simulink model "CML_Utility_Test"  (R2015a)
settings: Solver=ode4  SolverMode=MultiTasking  StartTime=0.0  StopTime=inf  FixedStep=BKIN_STEP_TIME  RelTol=1e-3
StartFcn:
  |  warndlg('Dexterit-E models cannot run under simulation. Please compile your model and run it from within Dexterit-E.');set_param(bdroot,'SimulationCommand','stop')
model workspace (MAT data in the model file):
  BKIN_STEP_TIME = 0.00025
  col_x = 1
  col_y = 2
  E_STAY_CENTER = 2
  INIT_COLOR = 5
  START_TARGET = 2
  MAX_REACH_TIME = 11
  DELAY_POST_TRIAL = 12
  BKIN_KINEMATIC_FRAME_SIZE = 400
  E_NO_EVENT = 0
  CHOICE_COLOR = 6
  FIXED_TARGET = 3
  FIXED_TARGET_VAL = 4
  GAMBLE_TARGET = 5
  GAMBLE_TARGET_VAL1 = 6
  GAMBLE_TARGET_VAL2 = 7
  DELAY_TARGET_FIXED = 8
  DELAY_TARGET_RANDOM = 9
  VWIDTH = 3
  VHEIGHT = 4
  TEXT = 8
  TEXT_COLOR = 9
  TEXT_HEIGHT = 10
  STROKE = 7
  TARGET_HOLD_TIME = 10
  E_HOLD_AT_FIXED_TARGET = 5
  E_HOLD_AT_GAMBLE_TARGET = 6
  K_SCORE_TARGET = 1
  E_CHOICES_ON = 3
  TRIAL_TYPE = 1
  E_PAUSE = 30
  E_EOT = 10
  CONTINUE = 2
  DELAY_CHOICE = 13
  E_WAIT = 4
  E_GO_TONE = 7
libraries: Video x4, General x3, slrtlib x3, KINARM_IO x2, KINARM_general x2, xpcnilib x2, simulink x1
CloseFcn:
  | rtwprivate ssgencode ModelCloseRequest b2lab2d
settings Model: ModifiedComment=chris -- Wed Feb 16 09:18:30 2005 -- Version 1.1384  ExtModeArmWhenConnect=off  ExtModeLogAll=off  LastModifiedBy=User
settings SolverCC: EnableConcurrentExecution=on  AutoInsertRateTranBlk=on
settings DataIOCC: LimitDataPoints=off  SignalLoggingSaveFormat=ModelDataLogs  SaveOutput=off  SaveTime=off  SignalLoggingName=sigsOut
settings OptimizationCC: BlockReduction=off  BooleanDataType=off  OptimizeBlockIOStorage=off  BufferReuse=off  GlobalBufferReuse=off  ExpressionFolding=off  ExpressionDepthLimit=2147483647  LocalBlockOutputs=off  InitFltsAndDblsToZero=on
settings DebuggingCC: SaveWithParameterizedLinksMsg=none  UnderspecifiedInitializationDetection=Classic  MergeDetectMultiDrivingBlocksExec=none  SignalResolutionControl=TryResolveAllWithWarning  MultiTaskDSMMsg=warning  FcnCallInpInsideContextMsg=UseLocalSettings  StateNameClashWarn=warning  StrictBusMsg=ErrorOnBusTreatedAsVector
settings HardwareCC: ProdIntDivRoundTo=Zero  ProdEndianess=LittleEndian  ProdLongLongMode=on  ProdHWDeviceType=Generic->32-bit x86 compatible  TargetHWDeviceType=32-bit Generic
settings SFSimCC: SimCustomHeaderCode="#include \"stdlib.h\""  SFSimEcho=off  SimParseCustomCode=off
settings RTWCC: SystemTargetFile=slrt.tlc  TemplateMakefile=slrt_default_tmf  Description=Simulink Real-Time  CustomSourceCode="#include \"stdlib.h\""  RTWCompilerOptimization=on
settings CodeAppCC: MaxIdLength=63
settings SimulinkRealTimeCC: TargetFcnLib=ansi_tfl_tmw.mat  GeneratePreprocessorConditionals=Disable all  xPCisDownloadable=off  xPCisDefaultEnv=off

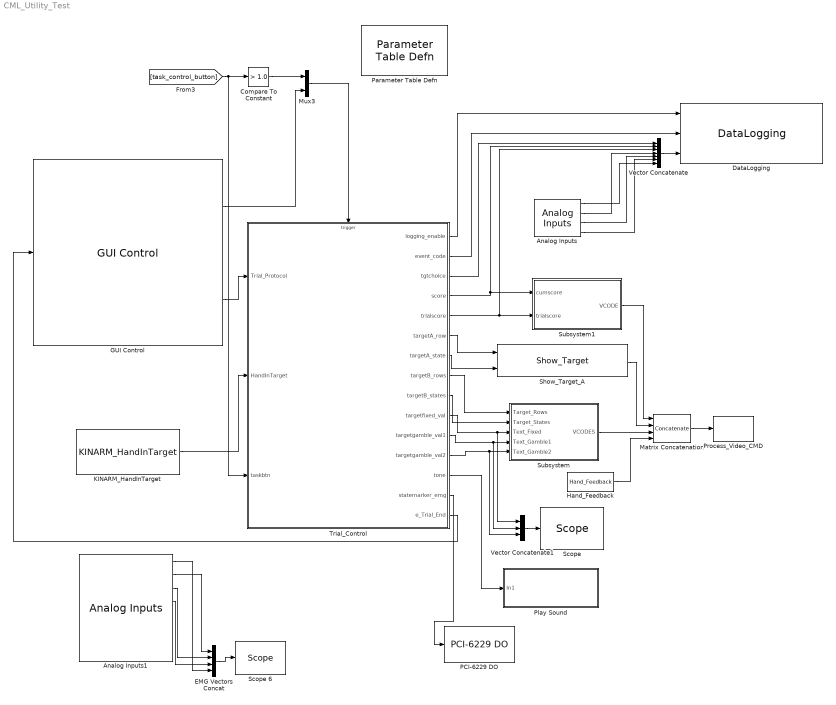
== system CML_Utility_Test ==
  Analog Inputs : KINARM_IO/Analog Inputs  channel=[17:20]  range=5  coupling=[0]  scantime6071e=1.28e-5  scantime6229=5e-6  sampletime=0.001  slot=-1  oscantime6071e=0
  Analog Inputs1 : KINARM_IO/Analog Inputs  channel=[17:24]  range=5  coupling=[0]  scantime6071e=1.28e-5  scantime6229=5e-6  sampletime=0.001  slot=-1  oscantime6071e=0
  Compare To Constant : simulink/Logic and Bit Operations/Compare To Constant  relop=>  const=1.0  OutDataTypeStr=boolean
  DataLogging : General/DataLogging  log_event_codes=on  log_analog_inputs=on  show_time_remaining=off  ecat_include=on
  EMG Vectors Concat : Concatenate  NumInputs=4
  GUI Control : General/GUI Control  task_version=1.0  show_repeat_trial_flag=off  use_custom_tp=off  target_type_str=Circle  Target_Type=1  XYcols=[1 2]  Vcols=3  Lcols=4  indices_padding=[0 0 0 0;0 0 0 0]  target_table_rows=64  load_table_rows=20  tp_table_rows=100
  Hand_Feedback : KINARM_general/Hand_Feedback  feedback_cntl_src=none
  KINARM_HandInTarget : KINARM_general/KINARM_HandInTarget  use_dominant_hand=on  target_type=Circle  num_states=1  attribcol1=[VWIDTH]  attribcol2=[0]  attribcol3=[0]  attribcol4=[0]  attribcol5=[0]
  Matrix Concatenation : Concatenate  NumInputs=4  Mode=Multidimensional array
  Mux3 : Mux  Inputs=2
  PCI-6229 DO : xpcnilib/Digital Output/M Series/PCI-6229 DO  channel=13  reset=[1]  initValue=[0]  sampletime=0.001  slot=-1
  Parameter Table Defn : General/Parameter Table Defn  ShowInLibBrowser=0
  Play Sound : Subsystem
  Process_Video_CMD : Video/Process_Video_CMD  video_delay=0
  "Scope " : slrtlib/Displays and Logging/Scope   scopeno=2  scopetype=Target  autostart=on  viewmode=Numerical  formatstr='%15.6f'  grid=on  ylimits=[0,0]  nosamples=4000  noprepostsamples=0  interleave=1  triggermode=FreeRun  triggersignal=1  trigsignalfromport=off  triggerlevel=0.0  triggerslope=Either  triggerscope=1  triggersample=0  filename=data.dat  mode=Lazy  writesize=512  autorestart=off  dynamicfilemode=off  maxwritefilesize=512*1024^2
  Scope 6 : slrtlib/Displays and Logging/Scope   scopeno=3  scopetype=Target  autostart=on  viewmode=Numerical  formatstr='%15.6f'  grid=on  ylimits=[0,0]  nosamples=250  noprepostsamples=0  interleave=1  triggermode=FreeRun  triggersignal=1  trigsignalfromport=off  triggerlevel=0.0  triggerslope=Either  triggerscope=1  triggersample=0  filename=data.dat  mode=Lazy  writesize=512  autorestart=off  dynamicfilemode=off  maxwritefilesize=512*1024^2
  Show_Target_A : Video/Show_Target  target_type=Circle  num_states=1  attribcol1=[INIT_COLOR 0 0 VWIDTH]  attribcol2=[0 0 0 0]  attribcol3=[0 0 0 0]  attribcol4=[0 0 0 0]  attribcol5=[0 0 0 0]  stateindices_padding=[0 0 0 0 0 0 0;0 0 0 0 0 0 0;0 0 0 0 0 0 0;0 0 0 0 0 0 0;0 0 0 0 0 0 0]  source=dialog  opacity=100  target_display=Both subject and operator displays  num_col=4
  Subsystem : Subsystem
  Subsystem1 : Subsystem
  Trial_Control : Stateflow chart  TreatAsAtomicUnit=on
  Vector Concatenate : Concatenate  NumInputs=7
  Vector Concatenate1 : Concatenate  NumInputs=3
  wires:
  KINARM_HandInTarget/1 -> Trial_Control/2(HandInTarget)
  Show_Target_A/1 -> Matrix Concatenation/2
  GUI Control/2 -> Trial_Control/1(Trial_Protocol)
  Trial_Control/15(e_Trial_End) -> GUI Control/1
  GUI Control/1 -> Mux3/2
  Trial_Control/7(targetA_state) -> Show_Target_A/2
  Trial_Control/6(targetA_row) -> Show_Target_A/1
  Matrix Concatenation/1 -> Process_Video_CMD/1
  Hand_Feedback/1 -> Matrix Concatenation/4
  Trial_Control/1(logging_enable) -> DataLogging/1
  Trial_Control/2(event_code) -> DataLogging/2
  Trial_Control/8(targetB_rows) -> Subsystem/1(Target_Rows)
  Trial_Control/9(targetB_states) -> Subsystem/2(Target_States)
  Trial_Control/10(targetfixed_val) -> Vector Concatenate1/1, Subsystem/3(Text_Fixed)
  Trial_Control/11(targetgamble_val1) -> Vector Concatenate1/2, Subsystem/4(Text_Gamble1)
  Trial_Control/12(targetgamble_val2) -> Vector Concatenate1/3, Subsystem/5(Text_Gamble2)
  Subsystem/1(VCODES) -> Matrix Concatenation/3
  Trial_Control/3(tgtchoice) -> Vector Concatenate/1
  Vector Concatenate/1 -> DataLogging/3
  Trial_Control/4(score) -> Vector Concatenate/2, Subsystem1/1(cumscore)
  Trial_Control/5(trialscore) -> Vector Concatenate/3, Subsystem1/2(trialscore)
  Subsystem1/1(VCODE) -> Matrix Concatenation/1
  Trial_Control/13(tone) -> Play Sound/1(In1)
  Vector Concatenate1/1 -> "Scope "/1
  [task_control_button] -> Trial_Control/3(taskbtn), Compare To Constant/1
  Mux3/1 -> Trial_Control/Trigger
  Compare To Constant/1 -> Mux3/1
  EMG Vectors Concat/1 -> Scope 6/1
  Analog Inputs1/1 -> EMG Vectors Concat/4
  Analog Inputs1/4 -> EMG Vectors Concat/3
  Analog Inputs1/2 -> EMG Vectors Concat/1
  Analog Inputs1/3 -> EMG Vectors Concat/2
  Analog Inputs/2 -> Vector Concatenate/4
  Analog Inputs/3 -> Vector Concatenate/5
  Analog Inputs/4 -> Vector Concatenate/6
  Analog Inputs/1 -> Vector Concatenate/7
  Trial_Control/14(statemarker_emg) -> PCI-6229 DO/1

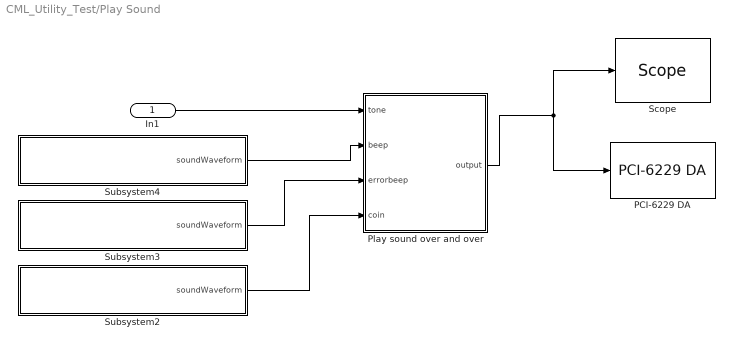
== system CML_Utility_Test/Play Sound ==
  In1 : Inport
  PCI-6229 DA : xpcnilib/D//A/M Series/PCI-6229 DA  channel=[1]  reset=[1]  initValue=[0]  sampletime=-1  slot=-1
  Play sound over and over : MATLAB Function  TreatAsAtomicUnit=on
  "Scope " : slrtlib/Displays and Logging/Scope   scopeno=1  scopetype=Target  autostart=on  viewmode=Graphical redraw  formatstr='%15.6f'  grid=on  ylimits=[0,0]  nosamples=4000  noprepostsamples=0  interleave=1  triggermode=FreeRun  triggersignal=1  trigsignalfromport=off  triggerlevel=0.0  triggerslope=Either  triggerscope=1  triggersample=0  filename=data.dat  mode=Lazy  writesize=512  autorestart=off  dynamicfilemode=off  maxwritefilesize=512*1024^2
  Subsystem2 : Subsystem  mask(Load Waveform Into Variable){fileName=coin}
      mask prompts: fileName "Name of .mat Data File (must be in current directory)"
      mask help: This block will load the .MAT file specified in the dialog, and put the first variable into a GoTo called 'soundWaveform'.
      mask init:
      | filenameFromMask = get_param(gcb, 'fileName');
      | 
      | try 
      | 	dataFromFile = load(filenameFromMask);
      | 	names = fieldnames(dataFromFile);
      | 	soundDataFromFile = dataFromFile.(names{1});
      | 	display(['Sound waveform from file ''' filenameFromMask ''' loaded.']);
      | catch ME
      | 	display(ME.message)
      | end
      mask Help:
      | Enter the name a .MAT file containing a single vector or matrix. The .MAT file must be located in the current directory.
      | 
      | The first variable from the .MAT file will be put into a Goto called 'soundWaveform'.
      mask Display: disp(['Load waveform from ''' filenameFromMask ''''])
  Subsystem3 : Subsystem  mask(Load Waveform Into Variable){fileName=errorbeep}
      mask prompts: fileName "Name of .mat Data File (must be in current directory)"
      mask help: This block will load the .MAT file specified in the dialog, and put the first variable into a GoTo called 'soundWaveform'.
      mask init: same as CML_Utility_Test/Play Sound/Subsystem2
      mask Help:
      | Enter the name a .MAT file containing a single vector or matrix. The .MAT file must be located in the current directory.
      | 
      | The first variable from the .MAT file will be put into a Goto called 'soundWaveform'.
      mask Display: disp(['Load waveform from ''' filenameFromMask ''''])
  Subsystem4 : Subsystem  mask(Load Waveform Into Variable){fileName=beep1khz}
      mask prompts: fileName "Name of .mat Data File (must be in current directory)"
      mask help: This block will load the .MAT file specified in the dialog, and put the first variable into a GoTo called 'soundWaveform'.
      mask init: same as CML_Utility_Test/Play Sound/Subsystem2
      mask Help:
      | Enter the name a .MAT file containing a single vector or matrix. The .MAT file must be located in the current directory.
      | 
      | The first variable from the .MAT file will be put into a Goto called 'soundWaveform'.
      mask Display: disp(['Load waveform from ''' filenameFromMask ''''])
  wires:
  Play sound over and over/1(output) -> PCI-6229 DA/1, "Scope "/1
  Subsystem3/1(soundWaveform) -> Play sound over and over/3(errorbeep)
  Subsystem4/1(soundWaveform) -> Play sound over and over/2(beep)
  In1/1 -> Play sound over and over/1(tone)
  Subsystem2/1(soundWaveform) -> Play sound over and over/4(coin)

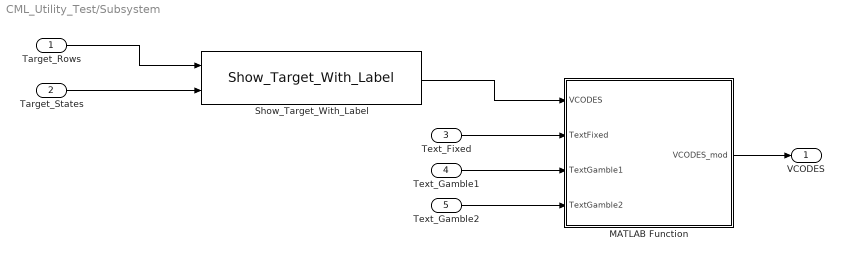
== system CML_Utility_Test/Subsystem ==
  Target_Rows : Inport
  Target_States : Inport  Port=2
  Text_Fixed : Inport  Port=3
  Text_Gamble1 : Inport  Port=4
  Text_Gamble2 : Inport  Port=5
  MATLAB Function : MATLAB Function  TreatAsAtomicUnit=on
  Show_Target_With_Label : Video/Show_Target_With_Label  target_type=Rectangle  num_states=2  attribcol1=[0 INIT_COLOR STROKE VWIDTH VHEIGHT 0 TEXT TEXT_COLOR TEXT_HEIGHT]  attribcol2=[CHOICE_COLOR INIT_COLOR STROKE VWIDTH VHEIGHT 0 TEXT TEXT_COLOR TEXT_HEIGHT]  attribcol3=[0 0 0 0 0 0 0 0 0]  attribcol4=[0 0 0 0 0 0 0 0 0]  attribcol5=[0 0 0 0 0 0 0 0 0]  stateindices_padding=[0 0;0 0;0 0;0 0;0 0]  source=dialog  opacity=100  target_display=Both subject and operator displays
  VCODES : Outport
  wires:
  MATLAB Function/1(VCODES_mod) -> VCODES/1
  Show_Target_With_Label/1 -> MATLAB Function/1(VCODES)
  Target_Rows/1 -> Show_Target_With_Label/1
  Target_States/1 -> Show_Target_With_Label/2
  Text_Fixed/1 -> MATLAB Function/2(TextFixed)
  Text_Gamble1/1 -> MATLAB Function/3(TextGamble1)
  Text_Gamble2/1 -> MATLAB Function/4(TextGamble2)

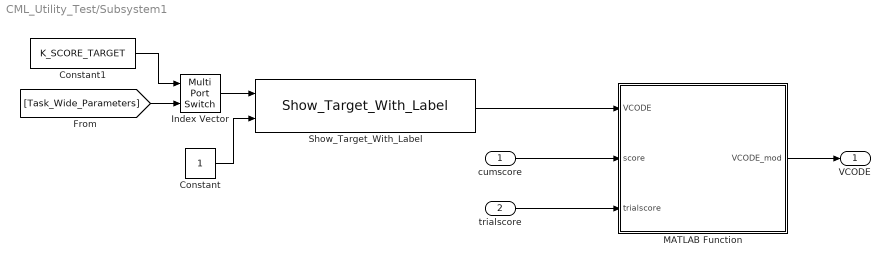
== system CML_Utility_Test/Subsystem1 ==
  cumscore : Inport
  trialscore : Inport  Port=2
  Constant : Constant
  Constant1 : Constant  Value=K_SCORE_TARGET
  Index Vector : MultiPortSwitch  Inputs=1
  MATLAB Function : MATLAB Function  TreatAsAtomicUnit=on
  Show_Target_With_Label : Video/Show_Target_With_Label  target_type=Rectangle  num_states=1  attribcol1=[0 0 0 VWIDTH TEXT_HEIGHT 0 TEXT TEXT_COLOR TEXT_HEIGHT]  attribcol2=[0 0 0 0 0 0 0 0 0]  attribcol3=[0 0 0 0 0 0 0 0 0]  attribcol4=[0 0 0 0 0 0 0 0 0]  attribcol5=[0 0 0 0 0 0 0 0 0]  stateindices_padding=[0 0;0 0;0 0;0 0;0 0]  source=dialog  opacity=100  target_display=Both subject and operator displays
  VCODE : Outport
  wires:
  MATLAB Function/1(VCODE_mod) -> VCODE/1
  Show_Target_With_Label/1 -> MATLAB Function/1(VCODE)
  cumscore/1 -> MATLAB Function/2(score)
  trialscore/1 -> MATLAB Function/3(trialscore)
  [Task_Wide_Parameters] -> Index Vector/2
  Index Vector/1 -> Show_Target_With_Label/1
  Constant/1 -> Show_Target_With_Label/2
  Constant1/1 -> Index Vector/1

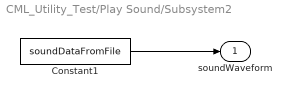
== system CML_Utility_Test/Play Sound/Subsystem2 ==
  Constant1 : Constant  Value=soundDataFromFile
  soundWaveform : Outport
  wires:
  Constant1/1 -> soundWaveform/1

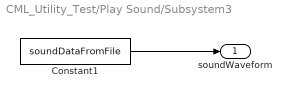
== system CML_Utility_Test/Play Sound/Subsystem3 ==
  Constant1 : Constant  Value=soundDataFromFile
  soundWaveform : Outport
  wires:
  Constant1/1 -> soundWaveform/1

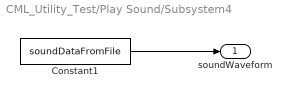
== system CML_Utility_Test/Play Sound/Subsystem4 ==
  Constant1 : Constant  Value=soundDataFromFile
  soundWaveform : Outport
  wires:
  Constant1/1 -> soundWaveform/1

== stateflow chart CML_Utility_Test/Trial_Control ==
  settings: sampleTime=0.001
  state MainTrial
    state MovToStart/
      TrialType = Trial_Protocol[TRIAL_TYPE];
    state InitPauseTrial1/
      // Just want to pause for a little
      event_code = E_PAUSE;
      logging_enable = 0;
    state ShowStartTarget/
      // Turn on first target, set loading conditions, enable data logging, and wait for a specified time or until the hand is in the target.
      targetA_row = Trial_Protocol[START_TARGET];
      targetA_state = 1;
      tgtchoice = 0;
      trialscore = 0;
    state HoldStartTarget/
      // Log an event that target was reached, begin data logging, change the first target's state, and then wait for a specified time.
      // The wait time may have both a fixed and a random component. The hand must stay in the target for the full wait time.
      event_code = E_STAY_CENTER;
      tickCount = Trial_Protocol[DELAY_TARGET_FIXED] + Trial_Protocol[DELAY_TARGET_RANDOM] * rand() / RAND_MAX;
      tick = 0;
      logging_enable = 1;
    state ShowChoiceTargets/
      // Turn on second target and log an event indicating this has occurred. Then wait until the hand is the target or until a specified time has elapsed.
      event_code = E_CHOICES_ON;
      targetB_rows[1] = Trial_Protocol[FIXED_TARGET];
      targetB_rows[2] = Trial_Protocol[GAMBLE_TARGET];
      targetB_states[1] = 1;
      targetB_states[2] = 1;
      targetfixed_val = Trial_Protocol[FIXED_TARGET_VAL];
      targetgamble_val1 = Trial_Protocol[GAMBLE_TARGET_VAL1];
      targetgamble_val2 = Trial_Protocol[GAMBLE_TARGET_VAL2];
      tickCount = Trial_Protocol[MAX_REACH_TIME];
      statemarker_emg=0;
      //tone = 1;
      during:
      tick++;
    state Wait/
      // Wait for specified amount of time before allowed to make a choice
      event_code=E_WAIT;
      //tone = 1;
      waitTime = Trial_Protocol[DELAY_CHOICE];
      statemarker_emg=1;
      during:
      tick++;
    state LeftStartTarget/
      event_code = E_GO_TONE;
      targetA_state = 0; //turn off target when hand leaves
      tone=1;
      during:
      tick++;
    state StayAtFixedTarget/
      // Fixed target was chosen
      event_code = E_HOLD_AT_FIXED_TARGET;
      targetB_states[1] = 2;
      tickCount = Trial_Protocol[TARGET_HOLD_TIME];
      tgtchoice = 1;
      trialscore = targetfixed_val;
      score += trialscore;
      tone = 2;
    state StayAtGambleTarget/
      // Fixed target was chosen
      event_code = E_HOLD_AT_GAMBLE_TARGET;
      targetB_states[2] = 2;
      tickCount = Trial_Protocol[TARGET_HOLD_TIME];
      tgtchoice = 2;
      tmprand = (rand() / RAND_MAX);
      trialscore = targetgamble_val1*(tmprand >= 0.5) + targetgamble_val2*(tmprand < 0.5);
      score += trialscore;
      tone = 2;
    state EndOfTrial/
      // Set the post-trial delay.
      statemarker_emg=0;
      event_code = E_EOT;
      tickCount = Trial_Protocol[DELAY_POST_TRIAL];
    MovToStart -> InitPauseTrial1 [order 1] : [TrialType==2]
    MovToStart -> ShowStartTarget [order 2] : [TrialType==1]
    InitPauseTrial1 -> EndOfTrial : [taskbtn==2]
    ShowStartTarget -> HoldStartTarget : [HandInTarget[targetA_row] == 1]
    HoldStartTarget -> ShowStartTarget [order 2] : [HandInTarget[targetA_row] == 0]
    HoldStartTarget -> ShowChoiceTargets [order 1] : after(tickCount, e_clk)
    ShowChoiceTargets -> HoldStartTarget [order 2] : [HandInTarget[targetA_row]==0]
    ShowChoiceTargets -> Wait [order 1] : after(1,e_clk)
    ShowChoiceTargets -> EndOfTrial [order 3] : [tick >= tickCount]
    Wait -> EndOfTrial [order 2] : [HandInTarget[targetA_row]==0]
    Wait -> LeftStartTarget [order 1] : after(waitTime, e_clk)
    LeftStartTarget -> EndOfTrial [order 1] : [tick >= tickCount]
    LeftStartTarget -> StayAtFixedTarget [order 3] : [HandInTarget[targetB_rows[1]]==1]
    LeftStartTarget -> StayAtGambleTarget [order 2] : [HandInTarget[targetB_rows[2]]==1]
    StayAtFixedTarget -> EndOfTrial : after(tickCount, e_clk)
    StayAtGambleTarget -> EndOfTrial : after(tickCount, e_clk)
  state Initialize/
    // Both the targets and data logging are initially off.
    targetA_state = 0;
    targetB_states[1] = 0;
    targetB_states[2] = 0;
    logging_enable = 0;
    score = 0;
    tone = 0;
    TrialType = Trial_Protocol[TRIAL_TYPE];
    statemarker_emg=0;
  state Inter_Trial_State/
    // Turn off both targets, turn off data logging, reset the
    // event code, and send the e_Trial_End Stateflow event.
    event_code = 0;
    targetA_state = 0;
    targetB_states[1] = 0;
    targetB_states[2] = 0;
    logging_enable = 0;
    tone = 0;
    statemarker_emg=0;
    TrialType = Trial_Protocol[TRIAL_TYPE];
    e_Trial_End;
  (default) -> Initialize
  Initialize -> MovToStart
  Inter_Trial_State -> MovToStart : after(tickCount, e_clk)
  MainTrial -> Inter_Trial_State : e_ExitTrialNow/
      | tickCount = 1;
  EndOfTrial -> Inter_Trial_State : after(1,e_clk)
  data: logging_enable output boolean; Trial_Protocol input double size=50; HandInTarget input double; event_code output uint16 [0..] =0; tgtchoice output double; score output double; trialscore output double; targetA_row output [1..32]; targetA_state output double; targetB_rows output double size=2; targetB_states output double size=2; tickCount local double; RAND_MAX constant double =32767; targetfixed_val output double; targetgamble_val1 output double; targetgamble_val2 output double; tone output double; tick local double; tmprand local double; TrialType local double; taskbtn input double; waitTime local double; statemarker_emg output double
  data targetA_row settings: description=index of the row currently being used in the TargetTable
  events: e_btn input EITHER_EDGE_EVENT; e_clk input RISING_EDGE_EVENT; e_ExitTrialNow input EITHER_EDGE_EVENT; e_Trial_End output EITHER_EDGE_EVENT

== matlab function CML_Utility_Test/Subsystem/MATLAB Function ==
  data: VCODES input; VCODES_mod output; TextFixed input; TextGamble1 input; TextGamble2 input
function VCODES_mod = fcn(VCODES, TextFixed, TextGamble1, TextGamble2)
%#codegen

%we have to replace the generic text with the desired text for this trial
%text goes into VCODE indexes 15-64 as numeric ASCII values

%    CR = 13
%    LF = 10
% space = 32
%     $ = 36
%   0-9 = 48-57
%     . = 46
%  cent = 162  %extended ASCII/16 bit unicode; This is not available in Dex

%VCODES_mod = VCODES;

%we cannot write out 3 lines of text in a single VCODE, so we will have to
%use 4 VCODES:
%  1: Fixed target + label
%  2: Gamble target + "or"
%  3: Gamble value 1, (x,y-label_height*1.5)
%  4: Gamble value 2, (x,y+label_height*1.5)

VCODES_mod = [VCODES(1,:); repmat(VCODES(2,:),3,1)];
VCODES_mod(3,4) = VCODES_mod(2,4)+VCODES_mod(2,66)*1.5; %set the y pos for the gamble1 val text
VCODES_mod(4,4) = VCODES_mod(2,4)-VCODES_mod(2,66)*1.5; %set the y pos for the gamble2 val text
VCODES_mod(3,6) = VCODES_mod(3,5); %set the line color to match the fill color, and the stroke width to zero
VCODES_mod(3,7) = 0;
VCODES_mod(4,6) = VCODES_mod(4,5); %set the line color to match the fill color, and the stroke width to zero
VCODES_mod(4,7) = 0;
%VCODES_mod(3,9) = 0; %set the target to be transparent
VCODES_mod(3,10) = VCODES_mod(3,10)/2; %reduce the target width
VCODES_mod(4,10) = VCODES_mod(4,10)/2; %reduce the target width
VCODES_mod(3,11) = VCODES_mod(3,66); %set the target height to match the text height
VCODES_mod(4,11) = VCODES_mod(4,66); %set the target height to match the text height

textcentschar = ' c'; %' cents';
textc = double(char(textcentschar)); %word "text"
%textcents = 162; %cents symbol?

textorchar = ' or ';
textor = double(char(textorchar));
%textor = [13 textor 13];

fixedtextout = [0 0 0 0 0 0 0 0];
gamble1textout = [0 0 0 0 0 0 0 0];
gamble2textout = [0 0 0 0 0 0 0 0];

%fix the rounding problem?
TextFixed = TextFixed+0.002;
TextGamble1 = TextGamble1+0.002;
TextGamble2 = TextGamble2+0.002;

%check if do dollars or cents
if (TextFixed > 1) && (TextGamble1 > 1) && (TextGamble2 > 1)
    dodollars = 1;
else
    dodollars = 0;
end


if dodollars == 1

%if TextFixed > 1
    %**TextFixed**
    dollars = int32(floor(double(TextFixed)));
    if (dollars >= 10) %double digit dollar value
        n1d = int32(floor(double(dollars)/10));
        n2d = dollars - n1d*10;
        textdollars = [int2char(int32(n1d)) int2char(int32(n2d))];
    else %single digit
        textdollars = int2char(int32(dollars));
    end
    
    cents = (TextFixed-double(dollars))*100;
    if (cents < 10)
        textcents = ['0' int2char(int32(cents))];
    else
        n1 = int32(floor(double(cents)/10));
        n2 = round(cents - n1*10);
        textcents = [int2char(int32(n1)) int2char(int32(n2))];
    end
    
    %need to translate text into ascii:
    fixedtextout = [36 double(textdollars) 46 double(textcents)];
    
    
    %**TextGamble1**
    dollars = int32(floor(double(TextGamble1)));
    if (dollars >= 10) %double digit dollar value
        n1d = int32(floor(double(dollars)/10));
        n2d = dollars - n1d*10;
        textdollars = [int2char(int32(n1d)) int2char(int32(n2d))];
    else %single digit
        textdollars = int2char(int32(dollars));
    end
    
    cents = (TextGamble1-double(dollars))*100;
    if (cents < 10)
        textcents = ['0' int2char(int32(cents))];
    else
        n1 = int32(floor(double(cents)/10));
        n2 = round(cents - n1*10);
        textcents = [int2char(int32(n1)) int2char(int32(n2))];
    end
    
    %need to translate text into ascii:
    gamble1textout = [36 double(textdollars) 46 double(textcents)];
    
    
    %**TextGamble2**
    dollars = int32(floor(double(TextGamble2)));
    if (dollars >= 10) %double digit dollar value
        n1d = int32(floor(double(dollars)/10));
        n2d = dollars - n1d*10;
        textdollars = [int2char(int32(n1d)) int2char(int32(n2d))];
    else %single digit
        textdollars = int2char(int32(dollars));
    end
    
    cents = (TextGamble2-double(dollars))*100;
    if (cents < 10)
        textcents = ['0' int2char(int32(cents))];
    else
        n1 = int32(floor(double(cents)/10));
        n2 = round(cents - n1*10);
        textcents = [int2char(int32(n1)) int2char(int32(n2))];
    end
    
    %need to translate text into ascii:
    gamble2textout = [36 double(textdollars) 46 double(textcents)];
    
    
else
    
    %**TextFixed**
    cents = int32(floor(double(TextFixed)*100));
    if (cents < 10)
        textcents = int2char(int32(cents));
    elseif cents < 100
        n1 = int32(floor(double(cents)/10));
        n2 = round(cents - n1*10);
        textcents = [int2char(int32(n1)) int2char(int32(n2))];
    else %we assume cents < 1000
        n1 = int32(floor(double(cents)/100));
        n2 = round(cents - n1*100);
        n2 = int32(floor(double(n2)/10));
        n3 = round(cents - n1*100 - n2*10);
        
        textcents = [int2char(int32(n1)) int2char(int32(n2)) int2char(int32(n3))];
    end
    
    fixedtextout = [double(textcents) textc];
    
    
    %**TextGamble1**
    cents = int32(floor(double(TextGamble1)*100));
    if (cents < 10)
        textcents = int2char(int32(cents));
    elseif cents < 100
        n1 = int32(floor(double(cents)/10));
        n2 = round(cents - n1*10);
        textcents = [int2char(int32(n1)) int2char(int32(n2))];
    else %we assume cents < 1000
        n1 = int32(floor(double(cents)/100));
        n2 = round(cents - n1*100);
        n2 = int32(floor(double(n2)/10));
        n3 = round(cents - n1*100 - n2*10);
        
        textcents = [int2char(int32(n1)) int2char(int32(n2)) int2char(int32(n3))];
    end
    
    gamble1textout = [double(textcents) textc];
    
    
    %**TextGamble2**
    cents = int32(floor(double(TextGamble2)*100));
    if (cents < 10)
        textcents = int2char(int32(cents));
    elseif cents < 100
        n1 = int32(floor(double(cents)/10));
        n2 = round(cents - n1*10);
        textcents = [int2char(int32(n1)) int2char(int32(n2))];
    else %we assume cents < 1000
        n1 = int32(floor(double(cents)/100));
        n2 = round(cents - n1*100);
        n2 = int32(floor(double(n2)/10));
        n3 = round(cents - n1*100 - n2*10);
        
        textcents = [int2char(int32(n1)) int2char(int32(n2)) int2char(int32(n3))];
    end
    
    gamble2textout = [double(textcents) textc];
    
    
end

% if TextGamble1 > 1
%     
%     dollars = int32(floor(double(TextGamble1)));
%     if (dollars >= 10) %double digit dollar value
%         n1d = int32(floor(double(dollars)/10));
%         n2d = dollars - n1d*10;
%         textdollars = [int2char(int32(n1d)) int2char(int32(n2d))];
%     else %single digit
%         textdollars = int2char(int32(dollars));
%     end
%     
%     cents = (TextGamble1-double(dollars))*100;
%     if (cents < 10)
%         textcents = ['0' int2char(int32(cents))];
%     else
%         n1 = int32(floor(double(cents)/10));
%         n2 = round(cents - n1*10);
%         textcents = [int2char(int32(n1)) int2char(int32(n2))];
%     end
%     
%     %need to translate text into ascii:
%     gamble1textout = [36 double(textdollars) 46 double(textcents)];
%     
% else
%     
%     cents = int32(floor(double(TextGamble1)*100));
%     if (cents < 10)
%         textcents = int2char(int32(cents));
%     else
%         n1 = int32(floor(double(cents)/10));
%         n2 = round(cents - n1*10);
%         textcents = [int2char(int32(n1)) int2char(int32(n2))];
%     end
%     
%     gamble1textout = [double(textcents) textc];
%     
% end
% 
% if TextGamble2 > 1
%     
%     dollars = int32(floor(double(TextGamble2)));
%     if (dollars >= 10) %double digit dollar value
%         n1d = int32(floor(double(dollars)/10));
%         n2d = dollars - n1d*10;
%         textdollars = [int2char(int32(n1d)) int2char(int32(n2d))];
%     else %single digit
%         textdollars = int2char(int32(dollars));
%     end
%     
%     cents = (TextGamble2-double(dollars))*100;
%     if (cents < 10)
%         textcents = ['0' int2char(int32(cents))];
%     else
%         n1 = int32(floor(double(cents)/10));
%         n2 = round(cents - n1*10);
%         textcents = [int2char(int32(n1)) int2char(int32(n2))];
%     end
%     
%     %need to translate text into ascii:
%     gamble2textout = [36 double(textdollars) 46 double(textcents)];
%     
% else
%     
%     cents = int32(floor(double(TextGamble2)*100));
%     if (cents < 10)
%         textcents = int2char(int32(cents));
%     else
%         n1 = int32(floor(double(cents)/10));
%         n2 = round(cents - n1*10);
%         textcents = [int2char(int32(n1)) int2char(int32(n2))];
%     end
%     
%     gamble2textout = [double(textcents) textc];
%     
% end

%gambletextout = [gamble1textout textor gamble2textout];

%we assume VCODE1 is the fixed target and VCODE2-4 is the gamble target
%we must make sure we won't overflow the VCODE: no more than 50 chars! so
%  clip off anything that overflows, and make sure to terminate the string
%  with the VCODE terminator code (0).

VCODES_mod(1,15:min([15+length(fixedtextout)-1,64])) = fixedtextout(1:min([length(fixedtextout),50])); %write out as many the characters as possible into the VCODE
VCODES_mod(1,min([15+length(fixedtextout)+1,64])) = 0;  %terminate the string!

VCODES_mod(2,15:min([15+length(textor)-1,64])) = textor(1:min([length(textor),50])); %write out as many the characters as possible into the VCODE
VCODES_mod(2,min([15+length(textor)+1,64])) = 0;  %terminate the string!

VCODES_mod(3,15:min([15+length(gamble1textout)-1,64])) = gamble1textout(1:min([length(gamble1textout),50])); %write out as many the characters as possible into the VCODE
VCODES_mod(3,min([15+length(gamble1textout)+1,64])) = 0;  %terminate the string!

VCODES_mod(4,15:min([15+length(gamble2textout)-1,64])) = gamble2textout(1:min([length(gamble2textout),50])); %write out as many the characters as possible into the VCODE
VCODES_mod(4,min([15+length(gamble2textout)+1,64])) = 0;  %terminate the string!

    
% dollars = int32(floor(double(score)/100));
% if (dollars >= 10) %double digit dollar value
%     n1d = int32(floor(double(dollars)/10));
%     n2d = dollars - n1d*10;
%     textdollars = [int2char(int32(n1d)) int2char(int32(n2d))];
% else %single digit
%     textdollars = int2char(int32(dollars));
% end
% 
% cents = score-dollars*100;
% if (cents < 10)
%     textcents = ['0' int2char(int32(cents))];
% else
%     n1 = int32(floor(double(cents)/10));
%     n2 = round(cents - n1*10);
%     textcents = [int2char(int32(n1)) int2char(int32(n2))];
% end
% 
% textout = [text1 textdollars text2 textcents text3];
% %need to translate text into ascii:
% textnum = double(textout); %this quickly casts each char into a number




function s = int2char(n)

n = mod(n,10); %make sure we only have 1 digit or we will get a weird character!

s = char(n+int32('0')); %// add the character

== matlab function CML_Utility_Test/Subsystem1/MATLAB Function ==
  data: VCODE input; VCODE_mod output; score input; trialscore input
function VCODE_mod = fcn(VCODE, score, trialscore)
%#codegen

%we have to replace the generic text with the desired text for this trial
%text goes into VCODE indexes 15-64 as numeric ASCII values

%    CR = 13
%    LF = 10
% space = 32
%     $ = 36
%   0-9 = 48-57
%     . = 46
%  cent = 162  %extended ASCII/16 bit unicode; Matlab recognizes it but may not work?

separatortext = '  /  ';
separatortext = double(char(separatortext));

VCODE_mod = VCODE;

%process the total cumulative score
% dollars = floor(score);
% dollars = double(char(num2str(dollars)));
% 
% cents = round((score - floor(score))*100);
% cents = double(char(num2str(cents)));
dollars = int32(floor(double(score)));
if (dollars >= 10) %double digit dollar value
    n1d = int32(floor(double(dollars)/10));
    n2d = dollars - n1d*10;
    textdollars = [int2char(int32(n1d)) int2char(int32(n2d))];
else %single digit
    textdollars = int2char(int32(dollars));
end

cents = (score-double(dollars))*100;
if (cents < 10)
    textcents = ['0' int2char(int32(cents))];
else
    n1 = int32(floor(double(cents)/10));
    n2 = round(cents - n1*10);
    textcents = [int2char(int32(n1)) int2char(int32(n2))];
end

%need to translate text into ascii:
scoretextout = [double(textdollars) 46 double(textcents)];


%process the current trial score
% dollars = floor(trialscore);
% dollars = double(char(num2str(dollars)));
% 
% cents = round((trialscore - floor(trialscore))*100);
% cents = double(char(num2str(cents)));
dollars = int32(floor(double(trialscore)));
if (dollars >= 10) %double digit dollar value
    n1d = int32(floor(double(dollars)/10));
    n2d = dollars - n1d*10;
    textdollars = [int2char(int32(n1d)) int2char(int32(n2d))];
else %single digit
    textdollars = int2char(int32(dollars));
end

cents = (trialscore-double(dollars))*100;
if (cents < 10)
    textcents = ['0' int2char(int32(cents))];
else
    n1 = int32(floor(double(cents)/10));
    n2 = round(cents - n1*10);
    textcents = [int2char(int32(n1)) int2char(int32(n2))];
end

%need to translate text into ascii:
trialscoretextout = [double(textdollars) 46 double(textcents)];

textout = [trialscoretextout separatortext scoretextout];


%we assume VCODE1 is the fixed target and VCODE2 is the gamble target
%we must make sure we won't overflow the VCODE: no more than 50 chars! so
%  clip off anything that overflows, and make sure to terminate the string
%  with the VCODE terminator code (0).

VCODE_mod(1,15:min([15+length(textout),64])) = textout(1:min([length(textout),50])); %write out as many the characters as possible into the VCODE
VCODE_mod(1,min([15+length(textout)+1,64])) = 0;  %terminate the string!



%we only want to display this to the experienter: 
%set VCODE(2):
% 0 - Do not show the target
% 1 - Show the target on the subject and operator displays
% 2 - Show the target on the subject display only
% 3 - Show the target on the operator display only
VCODE_mod(1,2) = 3;

    
% dollars = int32(floor(double(score)/100));
% if (dollars >= 10) %double digit dollar value
%     n1d = int32(floor(double(dollars)/10));
%     n2d = dollars - n1d*10;
%     textdollars = [int2char(int32(n1d)) int2char(int32(n2d))];
% else %single digit
%     textdollars = int2char(int32(dollars));
% end
% 
% cents = score-dollars*100;
% if (cents < 10)
%     textcents = ['0' int2char(int32(cents))];
% else
%     n1 = int32(floor(double(cents)/10));
%     n2 = round(cents - n1*10);
%     textcents = [int2char(int32(n1)) int2char(int32(n2))];
% end
% 
% textout = [text1 textdollars text2 textcents text3];
% %need to translate text into ascii:
% textnum = double(textout); %this quickly casts each char into a number





function s = int2char(n)

n = mod(n,10); %make sure we only have 1 digit or we will get a weird character!

s = char(n+int32('0')); %// add the character

== matlab function CML_Utility_Test/Play Sound/Play sound over and over ==
  data: tone input; output output; beep input; errorbeep input; coin input
function output = fcn(tone,beep,errorbeep,coin)
%#codegen

persistent t last_tone_state
if isempty(t), t = 0; end
if isempty(last_tone_state), last_tone_state = 0; end

trigger = last_tone_state ~= tone;
if trigger > 0
    last_tone_state = tone;
end

output = 0;		% default
if t == 0 && trigger > 0
	% start the playing of the sound.
	t = t + 1;
end

if tone == 1
    data = beep;
elseif tone == 2
    data = coin;
elseif tone == 3
    data = errorbeep;
else 
    t = 0;
    data = 0;
end

if t > 0
	output = data(t);
	if t == length(data)
		t = 0;
	else
		t = t + 1;
	end
end
